simulink model "ex3_sim1m"  (R2022b)
settings: Solver=ode45  StartTime=0.0  StopTime=4  MaxStep=0.0001  RelTol=1e-3
undefined symbols (not defined in the file): bit, denC, denP, numC, numP, r, Ts, umax
settings Model: Creator=loren  LastModifiedBy=loren
settings DataIOCC: ReturnWorkspaceOutputs=off

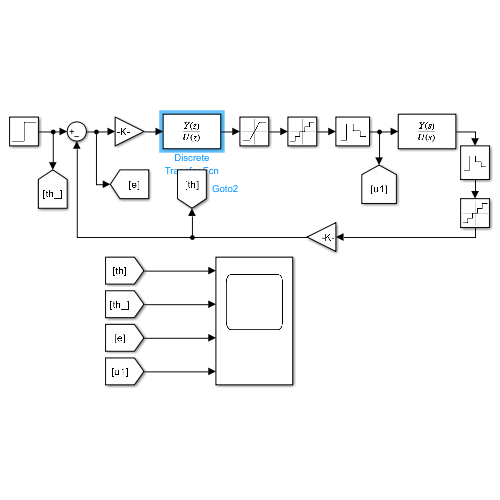
[thumbnail: Simulink's stored preview of the top-level diagram]
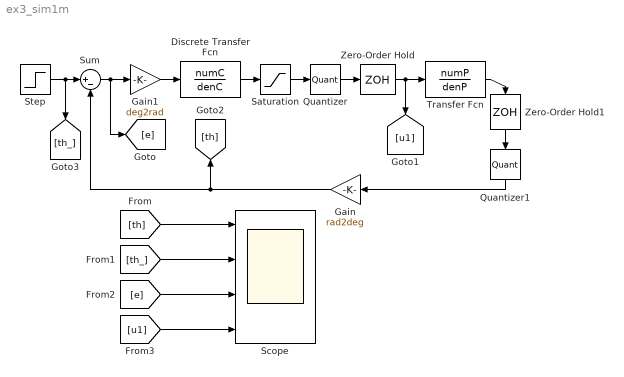
== system ex3_sim1m ==
  Discrete Transfer Fcn : DiscreteTransferFcn  Numerator=numC  Denominator=denC  SampleTime=Ts
  Gain : Gain  Gain=rad2deg
  Gain1 : Gain  Gain=deg2rad
  Quantizer : Quantizer  QuantizationInterval=2 * umax / 2^bit
  Quantizer1 : Quantizer  QuantizationInterval=pulse2rad
  Saturation : Saturate  UpperLimit=umax  LowerLimit=-umax
  Scope : Scope  NumInputPorts=4
  Step : Step  Time=r.t  After=r.A  SampleTime=0
  Sum : Sum  Inputs=|+-
  Transfer Fcn : TransferFcn  Numerator=numP  Denominator=denP
  Zero-Order Hold : ZeroOrderHold  SampleTime=Ts
  Zero-Order Hold1 : ZeroOrderHold  SampleTime=Ts
  wires:
  Step/1 -> [th_], Sum/1
  Discrete Transfer Fcn/1 -> Saturation/1
  Saturation/1 -> Quantizer/1
  Quantizer/1 -> Zero-Order Hold/1
  Zero-Order Hold/1 -> [u1], Transfer Fcn/1
  Transfer Fcn/1 -> Zero-Order Hold1/1
  Zero-Order Hold1/1 -> Quantizer1/1
  Sum/1 -> [e], Gain1/1
  Gain1/1 -> Discrete Transfer Fcn/1
  Gain/1 -> Sum/2, [th]
  [th] -> Scope/1
  [th_] -> Scope/2
  [e] -> Scope/3
  [u1] -> Scope/4
  Quantizer1/1 -> Gain/1
